simulink model "V2"  (R2024b)
settings: Solver=ode4  StartTime=0.0  StopTime=EXP.stop_time  FixedStep=EXP.physics_step  RelTol=1e-3
PostLoadFcn:
  | addpath(fullfile(fileparts(get_param(bdroot,'FileName')),'simulink_config')); v2_initialize_model(bdroot);
InitFcn:
  | addpath(fullfile(fileparts(get_param(bdroot,'FileName')),'simulink_config')); v2_initialize_model(bdroot);
model workspace (MAT data in the model file):
  CTRL.sample_time = 0.0025
  CTRL.position.Kp = [2.5 2.5 3.4]
  CTRL.position.Ki = [0 0 0]
  CTRL.position.Kd = [0 0 0]
  CTRL.position.integral_limit = [0.3 0.3 0.3]
  CTRL.position.output_limit = [10 10 100]
  CTRL.position.derivative_cutoff_hz = 10
  CTRL.position.velocity_ff.enable = 0
  CTRL.position.velocity_ff.cutoff_hz = 10
  CTRL.velocity.Kp = [3.5 3.5 8]
  CTRL.velocity.Ki = [0.12 0.12 2.5]
  CTRL.velocity.Kd = [0.08 0.08 0.07]
  CTRL.velocity.integral_limit = [10 10 10]
  CTRL.velocity.output_limit = [1000 1000 1000]
  CTRL.velocity.derivative_cutoff_hz = 10
  CTRL.velocity.gravity_comp.enable = 1
  CTRL.attitude.Kp = [10 10 4.5]
  CTRL.attitude.Ki = [0 0 0]
  CTRL.attitude.Kd = [0.05 0.05 0.01]
  CTRL.attitude.integral_limit = [0.2 0.2 0.2]
  CTRL.attitude.output_limit = [3.84 3.84 3.49]
  CTRL.attitude.derivative_cutoff_hz = 15
  CTRL.rate.Kp = [2.2 2.2 1.6]
  CTRL.rate.Ki = [0 0 0]
  CTRL.rate.Kd = [0.04 0.04 0.02]
  CTRL.rate.integral_limit = [0.4 0.4 0.4]
  CTRL.rate.output_limit = [4 4 3]
  CTRL.rate.derivative_cutoff_hz = 20
  CTRL.rate.gyroscopic_ff.enable = 1
  CTRL.force_limit = [30 30 100]
  CTRL.torque_limit = [5 5 4]
  CTRL.nominal.mass = 6
  CTRL.nominal.gravity = 9.80665
  CTRL.nominal.inertia = [0.2  0  0; 0  0.2  0; 0  0  0.2]
  CTRL.nominal.geometry.arm_length = 0.4
  CTRL.nominal.geometry.rotor_z = -0.015
  CTRL.nominal.geometry.radial_xy = [0.707106781187  -0.707106781187  -0.707106781187  0.707106781187; 0.707106781187  0.707106781187  -0.707106781187  -0.707106781187]
  CTRL.nominal.geometry.tangent = [0.707106781187  0.707106781187  -0.707106781187  -0.707106781187; -0.707106781187  0.707106781187  0.707106781187  -0.707106781187; 0  0  0  0]
  CTRL.nominal.geometry.spin = [-1 1 -1 1]
  CTRL.nominal.propeller.b_over_k = 0.01
  CTRL.nominal.propeller.reaction_torque_ratio = 0.01
  CTRL.nominal.propeller.max_thrust = 200
  CTRL.nominal.servo_limit = 1
  CTRL.allocator.yaw_split_cutoff_hz = 0.5
  CTRL.allocator.yaw_reaction_limit = 0.6
  CTRL.allocator.regularization = 1e-08
  CTRL.dob.enable = 1
  CTRL.dob.cutoff_rad_s = 2
  CTRL.dob.estimate_limit = [3 3 3]
  CTRL.moce.enable = 0
  CTRL.moce.gamma = [7e-06 7e-06 0.00015]
  CTRL.moce.initial_com = [0 0 0]
  CTRL.moce.offset_limit = [0.15 0.15 0.15]
  CTRL.moce.rate_limit = [0.02 0.02 0.02]
  CTRL.moce.min_force = 5
  CTRL.moce.estimate_z = 0
  CTRL.moce.min_horizontal_force = 0.1
  CTRL.moce.force_cutoff_rad_s = 2
  CTRL.moce.output_tau_s = 0.15
  EXP.command.position = [0 0 1]
  EXP.command.position_mode = 0
  EXP.command.position_sine_amplitude = [0 -10 0]
  EXP.command.position_sine_rad_s = [0 0.5 0]
  EXP.command.position_sine_phase = [0 0 0]
  EXP.command.position_start_s = 10
  EXP.command.attitude = [0 0 0]
  EXP.command.attitude_sine_enable = [0 0 0]
  EXP.command.attitude_sine_amplitude = [0.2 -0.2 -1]
  EXP.command.attitude_sine_rad_s = [0.4 0.4 0.2]
  EXP.command.attitude_sine_phase = [0 0 0]
  EXP.payload.mass = 0
  EXP.payload.position = [0 0 0]
  EXP.initial.position = [0 0 0]
  EXP.initial.velocity = [0 0 0]
  EXP.initial.attitude = [0 0 0]
  EXP.initial.body_rate = [0 0 0]
  EXP.seed = 1
  EXP.stop_time = 10
  EXP.physics_step = 0.00125
  PLANT.vehicle.mass = 6
  PLANT.vehicle.com = [0.01 0.005 0.001]
  PLANT.vehicle.inertia = [0.3  0  0; 0  0.3  0; 0  0  0.4]
  PLANT.gravity = 9.80665
  PLANT.geometry.arm_length = 0.4
  PLANT.geometry.rotor_z = -0.015
  PLANT.geometry.radial_xy = [0.707106781187  -0.707106781187  -0.707106781187  0.707106781187; 0.707106781187  0.707106781187  -0.707106781187  -0.707106781187]
  PLANT.geometry.tangent = [0.707106781187  0.707106781187  -0.707106781187  -0.707106781187; -0.707106781187  0.707106781187  0.707106781187  -0.707106781187; 0  0  0  0]
  PLANT.geometry.spin = [-1 1 -1 1]
  PLANT.propeller.b_over_k = 0.01
  PLANT.propeller.reaction_torque_ratio = 0.01
  PLANT.propeller.time_constant_s = 0.01
  PLANT.propeller.delay_s = 0
  PLANT.propeller.effectiveness = [0.8; 0.8; 0.8; 0.8]
  PLANT.propeller.max_thrust = 200
  PLANT.propeller.initial_thrust = [0; 0; 0; 0]
  PLANT.servo.time_constant_s = 0.0333333333333
  PLANT.servo.delay_s = 0
  PLANT.servo.dc_gain = 1
  PLANT.servo.limit_rad = 1
  PLANT.servo.initial_angle = [0; 0; 0; 0]
  PLANT.derived.mass = 6
  PLANT.derived.com = [0.01; 0.005; 0.001]
  PLANT.derived.inertia = [0.3  0  0; 0  0.3  0; 0  0  0.4]
  SENSOR.position.enable = 0
  SENSOR.position.noise_std = [0.00019 0.00022 0.00017]
  SENSOR.position.bias = [0 0 0]
  SENSOR.velocity.enable = 0
  SENSOR.velocity.noise_std = [0.00473 0.005 0.00368]
  SENSOR.velocity.bias = [0 0 0]
  SENSOR.attitude.enable = 0
  SENSOR.attitude.noise_std = [0.00071 0.00067 0.00044]
  SENSOR.attitude.bias = [0 0 0]
  SENSOR.gyro.enable = 0
  SENSOR.gyro.noise_std = [0.0236 0.0215 0.0174]
  SENSOR.gyro.bias = [0 0 0]
  SENSOR.delay_s = 0
settings Model: Creator=seosuk  LastModifiedBy=seosuk
settings DataIOCC: SaveOutput=off
settings DebuggingCC: AlgebraicLoopMsg=error

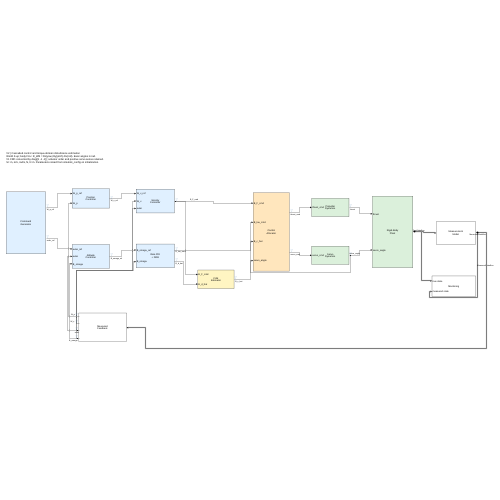
[thumbnail: Simulink's stored preview of the top-level diagram]
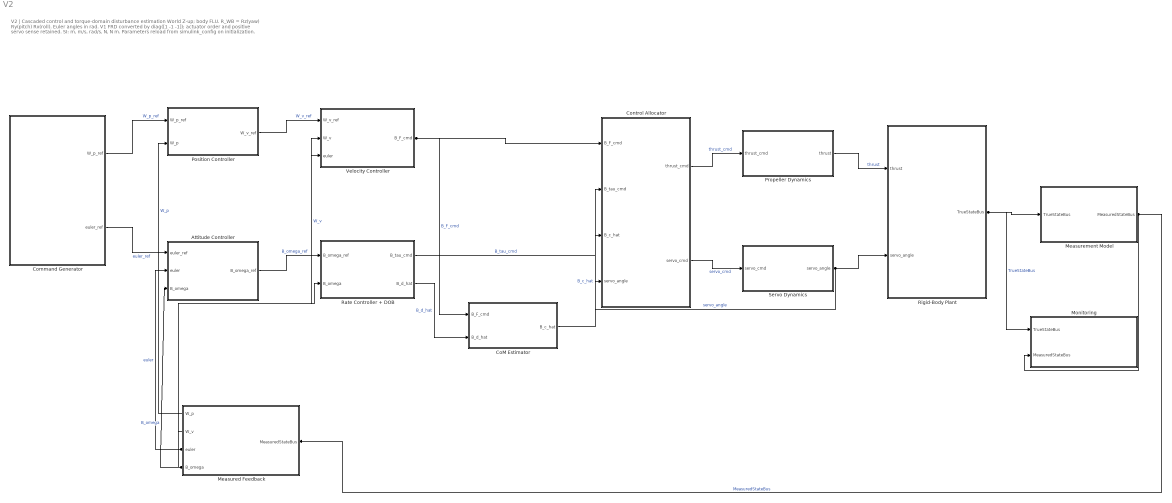
== system V2 ==
  note: V2 | Cascaded control and torque-domain disturbance estimation
      | World Z-up; body FLU. R_WB = Rz(yaw) Ry(pitch) Rx(roll). Euler angles in rad.
      | V1 FRD converted by diag([1 -1 -1]); actuator order and positive servo sense retained.
      | SI: m, m/s, rad/s, N, N m. Parameters reload from simulink_config on initialization.
  Attitude Controller : Subsystem
      mask Display:
      | disp(sprintf('Attitude\nController'));
      | port_label('input',1,'euler_ref');
      | port_label('input',2,'euler');
      | port_label('input',3,'B_omega');
  CoM Estimator : Subsystem
      mask Display:
      | disp(sprintf('CoM\nEstimator'));
      | port_label('input',1,'B_F_cmd');
      | port_label('input',2,'B_d_hat');
  Command Generator : Subsystem
      mask Display: disp(sprintf('Command\nGenerator'));
  Control Allocator : Subsystem
      mask Display:
      | disp(sprintf('Control\nAllocator'));
      | port_label('input',1,'B_F_cmd');
      | port_label('input',2,'B_tau_cmd');
      | port_label('input',3,'B_c_hat');
      | port_label('input',4,'servo_angle');
  Measured Feedback : Subsystem
      mask Display: disp(sprintf('Measured\nFeedback'));
  Measurement Model : Subsystem
      mask Display: disp(sprintf('Measurement\nModel'));
  Monitoring : Subsystem
      mask Display:
      | disp(sprintf('Monitoring'));
      | port_label('input',1,'true state');
      | port_label('input',2,'measured state');
  Position Controller : Subsystem
      mask Display:
      | disp(sprintf('Position\nController'));
      | port_label('input',1,'W_p_ref');
      | port_label('input',2,'W_p');
  Propeller Dynamics : Subsystem
      mask Display:
      | disp(sprintf('Propeller\nDynamics'));
      | port_label('input',1,'thrust_cmd');
  Rate Controller + DOB : Subsystem
      mask Display:
      | disp(sprintf('Rate PID\n+ DOB'));
      | port_label('input',1,'B_omega_ref');
      | port_label('input',2,'B_omega');
  Rigid-Body Plant : Subsystem
      mask Display:
      | disp(sprintf('Rigid-Body\nPlant'));
      | port_label('input',1,'thrust');
      | port_label('input',2,'servo_angle');
  Servo Dynamics : Subsystem
      mask Display:
      | disp(sprintf('Servo\nDynamics'));
      | port_label('input',1,'servo_cmd');
  Velocity Controller : Subsystem
      mask Display:
      | disp(sprintf('Velocity\nController'));
      | port_label('input',1,'W_v_ref');
      | port_label('input',2,'W_v');
      | port_label('input',3,'euler');
  wires:
  Command Generator/1(W_p_ref) -> Position Controller/1(W_p_ref)  "W_p_ref"
  Command Generator/2(euler_ref) -> Attitude Controller/1(euler_ref)  "euler_ref"
  Position Controller/1(W_v_ref) -> Velocity Controller/1(W_v_ref)  "W_v_ref"
  Velocity Controller/1(B_F_cmd) -> Control Allocator/1(B_F_cmd), CoM Estimator/1(B_F_cmd)  "B_F_cmd"
  Attitude Controller/1(B_omega_ref) -> Rate Controller + DOB/1(B_omega_ref)  "B_omega_ref"
  Rate Controller + DOB/1(B_tau_cmd) -> Control Allocator/2(B_tau_cmd)  "B_tau_cmd"
  Rate Controller + DOB/2(B_d_hat) -> CoM Estimator/2(B_d_hat)  "B_d_hat"
  CoM Estimator/1(B_c_hat) -> Control Allocator/3(B_c_hat)  "B_c_hat"
  Control Allocator/1(thrust_cmd) -> Propeller Dynamics/1(thrust_cmd)  "thrust_cmd"
  Control Allocator/2(servo_cmd) -> Servo Dynamics/1(servo_cmd)  "servo_cmd"
  Propeller Dynamics/1(thrust) -> Rigid-Body Plant/1(thrust)  "thrust"
  Servo Dynamics/1(servo_angle) -> Rigid-Body Plant/2(servo_angle), Control Allocator/4(servo_angle)  "servo_angle"
  Rigid-Body Plant/1(TrueStateBus) -> Measurement Model/1(TrueStateBus), Monitoring/1(TrueStateBus)  "TrueStateBus"
  Measurement Model/1(MeasuredStateBus) -> Monitoring/2(MeasuredStateBus), Measured Feedback/1(MeasuredStateBus)  "MeasuredStateBus"
  Measured Feedback/1(W_p) -> Position Controller/2(W_p)  "W_p"
  Measured Feedback/2(W_v) -> Velocity Controller/2(W_v)  "W_v"
  Measured Feedback/3(euler) -> Velocity Controller/3(euler), Attitude Controller/2(euler)  "euler"
  Measured Feedback/4(B_omega) -> Attitude Controller/3(B_omega), Rate Controller + DOB/2(B_omega)  "B_omega"

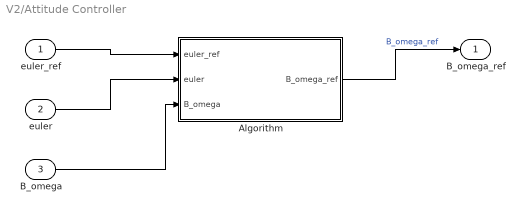
== system V2/Attitude Controller ==
  euler_ref : Inport  PortDimensions=[3 1]
  euler : Inport  Port=2  PortDimensions=[3 1]
  B_omega : Inport  Port=3  PortDimensions=[3 1]
  Algorithm : MATLAB Function  TreatAsAtomicUnit=on
  B_omega_ref : Outport
  wires:
  euler_ref/1 -> Algorithm/1(euler_ref)
  euler/1 -> Algorithm/2(euler)
  B_omega/1 -> Algorithm/3(B_omega)
  Algorithm/1(B_omega_ref) -> B_omega_ref/1  "B_omega_ref"

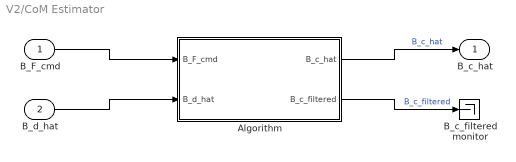
== system V2/CoM Estimator ==
  B_F_cmd : Inport  PortDimensions=[3 1]
  B_d_hat : Inport  Port=2  PortDimensions=[3 1]
  Algorithm : MATLAB Function  TreatAsAtomicUnit=on
  B_c_filtered monitor : Terminator
  B_c_hat : Outport
  wires:
  B_F_cmd/1 -> Algorithm/1(B_F_cmd)
  B_d_hat/1 -> Algorithm/2(B_d_hat)
  Algorithm/1(B_c_hat) -> B_c_hat/1  "B_c_hat"
  Algorithm/2(B_c_filtered) -> B_c_filtered monitor/1  "B_c_filtered"

== system V2/Command Generator ==
  Algorithm : MATLAB Function  TreatAsAtomicUnit=on
  Experiment time : Clock
  W_p_ref : Outport
  euler_ref : Outport  Port=2
  wires:
  Algorithm/1(W_p_ref) -> W_p_ref/1  "W_p_ref"
  Algorithm/2(euler_ref) -> euler_ref/1  "euler_ref"
  Experiment time/1 -> Algorithm/1(t)

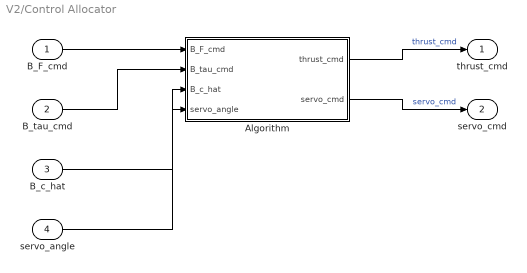
== system V2/Control Allocator ==
  B_F_cmd : Inport  PortDimensions=[3 1]
  B_tau_cmd : Inport  Port=2  PortDimensions=[3 1]
  B_c_hat : Inport  Port=3  PortDimensions=[3 1]
  servo_angle : Inport  Port=4  PortDimensions=[4 1]
  Algorithm : MATLAB Function  TreatAsAtomicUnit=on
  thrust_cmd : Outport
  servo_cmd : Outport  Port=2
  wires:
  B_F_cmd/1 -> Algorithm/1(B_F_cmd)
  B_tau_cmd/1 -> Algorithm/2(B_tau_cmd)
  B_c_hat/1 -> Algorithm/3(B_c_hat)
  servo_angle/1 -> Algorithm/4(servo_angle)
  Algorithm/1(thrust_cmd) -> thrust_cmd/1  "thrust_cmd"
  Algorithm/2(servo_cmd) -> servo_cmd/1  "servo_cmd"

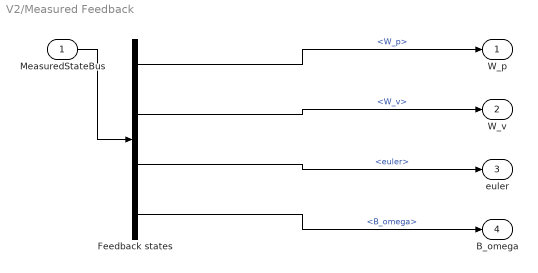
== system V2/Measured Feedback ==
  MeasuredStateBus : Inport
  Feedback states : BusSelector  OutputSignals=W_p,W_v,euler,B_omega
  W_p : Outport
  W_v : Outport  Port=2
  euler : Outport  Port=3
  B_omega : Outport  Port=4
  wires:
  MeasuredStateBus/1 -> Feedback states/1
  Feedback states/1 -> W_p/1  "<W_p>"
  Feedback states/2 -> W_v/1  "<W_v>"
  Feedback states/3 -> euler/1  "<euler>"
  Feedback states/4 -> B_omega/1  "<B_omega>"

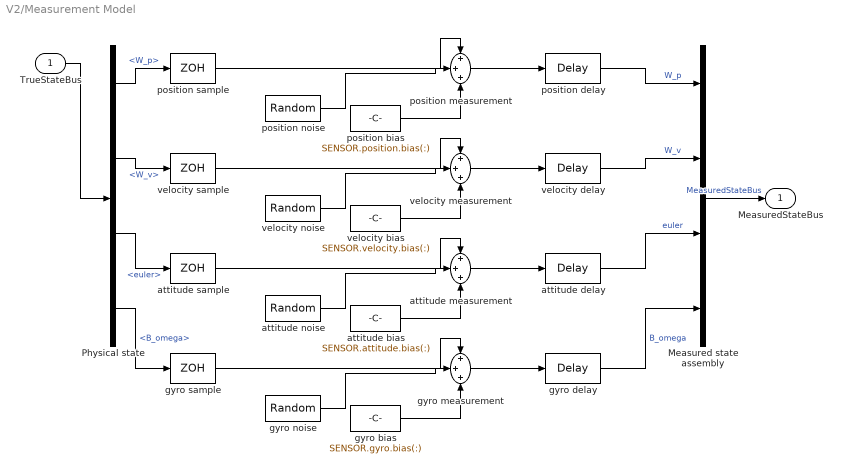
== system V2/Measurement Model ==
  TrueStateBus : Inport
  Measured state assembly : BusCreator  Inputs=4
  Physical state : BusSelector  OutputSignals=W_p,W_v,euler,B_omega
  attitude bias : Constant  Value=SENSOR.attitude.bias(:)
  attitude delay : TransportDelay  DelayTime=SENSOR.delay_s  TransDelayFeedthrough=on
  attitude measurement : Sum  Inputs=+++
  attitude noise : RandomNumber  Mean=[0;0;0]  Variance=double(SENSOR.attitude.enable)*SENSOR.attitude.noise_std(:).^2  Seed=EXP.seed+303  SampleTime=CTRL.sample_time
  attitude sample : ZeroOrderHold  SampleTime=CTRL.sample_time
  gyro bias : Constant  Value=SENSOR.gyro.bias(:)
  gyro delay : TransportDelay  DelayTime=SENSOR.delay_s  TransDelayFeedthrough=on
  gyro measurement : Sum  Inputs=+++
  gyro noise : RandomNumber  Mean=[0;0;0]  Variance=double(SENSOR.gyro.enable)*SENSOR.gyro.noise_std(:).^2  Seed=EXP.seed+404  SampleTime=CTRL.sample_time
  gyro sample : ZeroOrderHold  SampleTime=CTRL.sample_time
  position bias : Constant  Value=SENSOR.position.bias(:)
  position delay : TransportDelay  DelayTime=SENSOR.delay_s  TransDelayFeedthrough=on
  position measurement : Sum  Inputs=+++
  position noise : RandomNumber  Mean=[0;0;0]  Variance=double(SENSOR.position.enable)*SENSOR.position.noise_std(:).^2  Seed=EXP.seed+101  SampleTime=CTRL.sample_time
  position sample : ZeroOrderHold  SampleTime=CTRL.sample_time
  velocity bias : Constant  Value=SENSOR.velocity.bias(:)
  velocity delay : TransportDelay  DelayTime=SENSOR.delay_s  TransDelayFeedthrough=on
  velocity measurement : Sum  Inputs=+++
  velocity noise : RandomNumber  Mean=[0;0;0]  Variance=double(SENSOR.velocity.enable)*SENSOR.velocity.noise_std(:).^2  Seed=EXP.seed+202  SampleTime=CTRL.sample_time
  velocity sample : ZeroOrderHold  SampleTime=CTRL.sample_time
  MeasuredStateBus : Outport
  wires:
  TrueStateBus/1 -> Physical state/1
  Physical state/1 -> position sample/1  "<W_p>"
  position sample/1 -> position measurement/1
  position noise/1 -> position measurement/2
  position bias/1 -> position measurement/3
  position measurement/1 -> position delay/1
  position delay/1 -> Measured state assembly/1  "W_p"
  Physical state/2 -> velocity sample/1  "<W_v>"
  velocity sample/1 -> velocity measurement/1
  velocity noise/1 -> velocity measurement/2
  velocity bias/1 -> velocity measurement/3
  velocity measurement/1 -> velocity delay/1
  velocity delay/1 -> Measured state assembly/2  "W_v"
  Physical state/3 -> attitude sample/1  "<euler>"
  attitude sample/1 -> attitude measurement/1
  attitude noise/1 -> attitude measurement/2
  attitude bias/1 -> attitude measurement/3
  attitude measurement/1 -> attitude delay/1
  attitude delay/1 -> Measured state assembly/3  "euler"
  Physical state/4 -> gyro sample/1  "<B_omega>"
  gyro sample/1 -> gyro measurement/1
  gyro noise/1 -> gyro measurement/2
  gyro bias/1 -> gyro measurement/3
  gyro measurement/1 -> gyro delay/1
  gyro delay/1 -> Measured state assembly/4  "B_omega"
  Measured state assembly/1 -> MeasuredStateBus/1  "MeasuredStateBus"

== system V2/Monitoring ==
  note: Read-only diagnostics. All named control/actuator signals are logged to logsout.
      | Use Simulation Data Inspector or out.logsout. PID/nominal torque and filtered CoM
      | are logged inside their producing subsystems, with no diagnostic feedback.
  TrueStateBus : Inport
  MeasuredStateBus : Inport  Port=2
  Measured state : Scope
  True state : Scope
  wires:
  TrueStateBus/1 -> True state/1
  MeasuredStateBus/1 -> Measured state/1

== system V2/Position Controller ==
  W_p_ref : Inport  PortDimensions=[3 1]
  W_p : Inport  Port=2  PortDimensions=[3 1]
  Algorithm : MATLAB Function  TreatAsAtomicUnit=on
  W_v_ref : Outport
  wires:
  W_p_ref/1 -> Algorithm/1(W_p_ref)
  W_p/1 -> Algorithm/2(W_p)
  Algorithm/1(W_v_ref) -> W_v_ref/1  "W_v_ref"

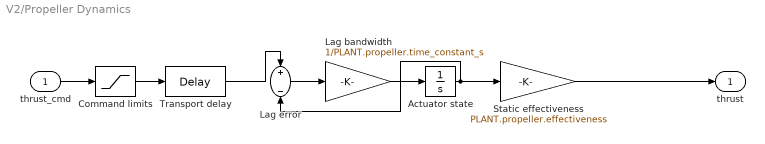
== system V2/Propeller Dynamics ==
  thrust_cmd : Inport  PortDimensions=[4 1]
  Actuator state : Integrator  InitialCondition=PLANT.propeller.initial_thrust
  Command limits : Saturate  UpperLimit=PLANT.propeller.max_thrust  LowerLimit=0
  Lag bandwidth : Gain  Gain=1/PLANT.propeller.time_constant_s
  Lag error : Sum  Inputs=+-
  Static effectiveness : Gain  Gain=PLANT.propeller.effectiveness
  Transport delay : TransportDelay  DelayTime=PLANT.propeller.delay_s  TransDelayFeedthrough=on
  thrust : Outport
  wires:
  thrust_cmd/1 -> Command limits/1
  Command limits/1 -> Transport delay/1
  Transport delay/1 -> Lag error/1
  Actuator state/1 -> Lag error/2, Static effectiveness/1
  Lag error/1 -> Lag bandwidth/1
  Lag bandwidth/1 -> Actuator state/1
  Static effectiveness/1 -> thrust/1

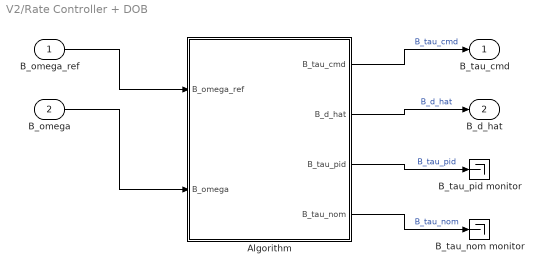
== system V2/Rate Controller + DOB ==
  B_omega_ref : Inport  PortDimensions=[3 1]
  B_omega : Inport  Port=2  PortDimensions=[3 1]
  Algorithm : MATLAB Function  TreatAsAtomicUnit=on
  B_tau_nom monitor : Terminator
  B_tau_pid monitor : Terminator
  B_tau_cmd : Outport
  B_d_hat : Outport  Port=2
  wires:
  B_omega_ref/1 -> Algorithm/1(B_omega_ref)
  B_omega/1 -> Algorithm/2(B_omega)
  Algorithm/1(B_tau_cmd) -> B_tau_cmd/1  "B_tau_cmd"
  Algorithm/2(B_d_hat) -> B_d_hat/1  "B_d_hat"
  Algorithm/3(B_tau_pid) -> B_tau_pid monitor/1  "B_tau_pid"
  Algorithm/4(B_tau_nom) -> B_tau_nom monitor/1  "B_tau_nom"

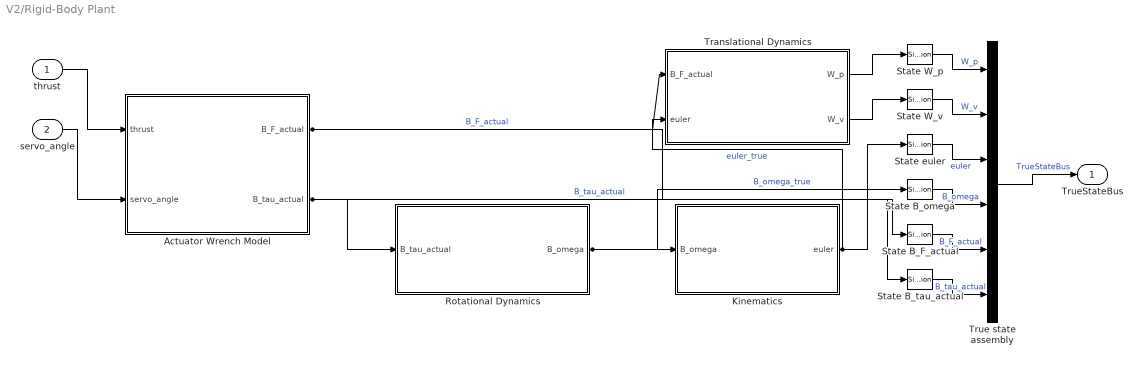
== system V2/Rigid-Body Plant ==
  thrust : Inport
  servo_angle : Inport  Port=2
  Actuator Wrench Model : Subsystem
  Kinematics : Subsystem
  Rotational Dynamics : Subsystem
  State B_F_actual : SignalConversion  OverrideOpt=off
  State B_omega : SignalConversion  OverrideOpt=off
  State B_tau_actual : SignalConversion  OverrideOpt=off
  State W_p : SignalConversion  OverrideOpt=off
  State W_v : SignalConversion  OverrideOpt=off
  State euler : SignalConversion  OverrideOpt=off
  Translational Dynamics : Subsystem
  True state assembly : BusCreator  Inputs=6
  TrueStateBus : Outport
  wires:
  thrust/1 -> Actuator Wrench Model/1(thrust)
  servo_angle/1 -> Actuator Wrench Model/2(servo_angle)
  Actuator Wrench Model/1(B_F_actual) -> Translational Dynamics/1(B_F_actual), State B_F_actual/1  "B_F_actual"
  Actuator Wrench Model/2(B_tau_actual) -> Rotational Dynamics/1(B_tau_actual), State B_tau_actual/1  "B_tau_actual"
  Rotational Dynamics/1(B_omega) -> Kinematics/1(B_omega), State B_omega/1  "B_omega_true"
  Kinematics/1(euler) -> Translational Dynamics/2(euler), State euler/1  "euler_true"
  Translational Dynamics/1(W_p) -> State W_p/1
  State W_p/1 -> True state assembly/1  "W_p"
  Translational Dynamics/2(W_v) -> State W_v/1
  State W_v/1 -> True state assembly/2  "W_v"
  State euler/1 -> True state assembly/3  "euler"
  State B_omega/1 -> True state assembly/4  "B_omega"
  State B_F_actual/1 -> True state assembly/5  "B_F_actual"
  State B_tau_actual/1 -> True state assembly/6  "B_tau_actual"
  True state assembly/1 -> TrueStateBus/1  "TrueStateBus"

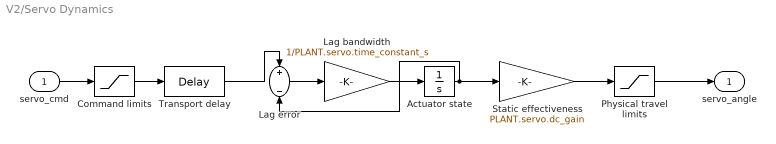
== system V2/Servo Dynamics ==
  servo_cmd : Inport  PortDimensions=[4 1]
  Actuator state : Integrator  InitialCondition=PLANT.servo.initial_angle
  Command limits : Saturate  UpperLimit=PLANT.servo.limit_rad  LowerLimit=-PLANT.servo.limit_rad
  Lag bandwidth : Gain  Gain=1/PLANT.servo.time_constant_s
  Lag error : Sum  Inputs=+-
  Physical travel limits : Saturate  UpperLimit=PLANT.servo.limit_rad  LowerLimit=-PLANT.servo.limit_rad
  Static effectiveness : Gain  Gain=PLANT.servo.dc_gain
  Transport delay : TransportDelay  DelayTime=PLANT.servo.delay_s  TransDelayFeedthrough=on
  servo_angle : Outport
  wires:
  servo_cmd/1 -> Command limits/1
  Command limits/1 -> Transport delay/1
  Transport delay/1 -> Lag error/1
  Actuator state/1 -> Lag error/2, Static effectiveness/1
  Lag error/1 -> Lag bandwidth/1
  Lag bandwidth/1 -> Actuator state/1
  Static effectiveness/1 -> Physical travel limits/1
  Physical travel limits/1 -> servo_angle/1

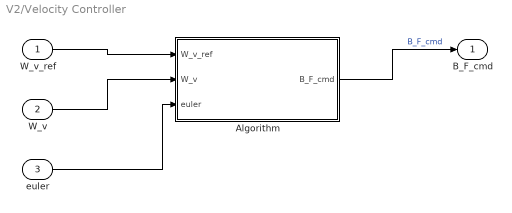
== system V2/Velocity Controller ==
  W_v_ref : Inport  PortDimensions=[3 1]
  W_v : Inport  Port=2  PortDimensions=[3 1]
  euler : Inport  Port=3  PortDimensions=[3 1]
  Algorithm : MATLAB Function  TreatAsAtomicUnit=on
  B_F_cmd : Outport
  wires:
  W_v_ref/1 -> Algorithm/1(W_v_ref)
  W_v/1 -> Algorithm/2(W_v)
  euler/1 -> Algorithm/3(euler)
  Algorithm/1(B_F_cmd) -> B_F_cmd/1  "B_F_cmd"

== system V2/Rigid-Body Plant/Actuator Wrench Model ==
  thrust : Inport  PortDimensions=[4 1]
  servo_angle : Inport  Port=2  PortDimensions=[4 1]
  Algorithm : MATLAB Function  TreatAsAtomicUnit=on
  B_F_actual : Outport
  B_tau_actual : Outport  Port=2
  wires:
  thrust/1 -> Algorithm/1(thrust)
  servo_angle/1 -> Algorithm/2(servo_angle)
  Algorithm/1(B_F_actual) -> B_F_actual/1  "B_F_actual"
  Algorithm/2(B_tau_actual) -> B_tau_actual/1  "B_tau_actual"

== system V2/Rigid-Body Plant/Kinematics ==
  B_omega : Inport
  Euler angle rates : Subsystem
  Euler attitude : Integrator  InitialCondition=EXP.initial.attitude(:)
  euler : Outport
  wires:
  B_omega/1 -> Euler angle rates/2(B_omega)
  Euler angle rates/1(euler_dot) -> Euler attitude/1
  Euler attitude/1 -> Euler angle rates/1(euler), euler/1

== system V2/Rigid-Body Plant/Rotational Dynamics ==
  B_tau_actual : Inport
  Body rate : Integrator  InitialCondition=EXP.initial.body_rate(:)
  Euler rigid body equation : Subsystem
  B_omega : Outport
  wires:
  B_tau_actual/1 -> Euler rigid body equation/1(B_tau_actual)
  Euler rigid body equation/1(B_omega_dot) -> Body rate/1
  Body rate/1 -> Euler rigid body equation/2(B_omega), B_omega/1

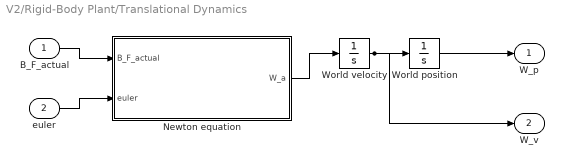
== system V2/Rigid-Body Plant/Translational Dynamics ==
  B_F_actual : Inport
  euler : Inport  Port=2
  Newton equation : Subsystem
  World position : Integrator  InitialCondition=EXP.initial.position(:)
  World velocity : Integrator  InitialCondition=EXP.initial.velocity(:)
  W_p : Outport
  W_v : Outport  Port=2
  wires:
  B_F_actual/1 -> Newton equation/1(B_F_actual)
  euler/1 -> Newton equation/2(euler)
  Newton equation/1(W_a) -> World velocity/1
  World velocity/1 -> World position/1, W_v/1
  World position/1 -> W_p/1

== system V2/Rigid-Body Plant/Kinematics/Euler angle rates ==
  euler : Inport  PortDimensions=[3 1]
  B_omega : Inport  Port=2  PortDimensions=[3 1]
  Algorithm : MATLAB Function  TreatAsAtomicUnit=on
  euler_dot : Outport
  wires:
  euler/1 -> Algorithm/1(euler)
  B_omega/1 -> Algorithm/2(B_omega)
  Algorithm/1(euler_dot) -> euler_dot/1  "euler_dot"

== system V2/Rigid-Body Plant/Rotational Dynamics/Euler rigid body equation ==
  B_tau_actual : Inport  PortDimensions=[3 1]
  B_omega : Inport  Port=2  PortDimensions=[3 1]
  Algorithm : MATLAB Function  TreatAsAtomicUnit=on
  B_omega_dot : Outport
  wires:
  B_tau_actual/1 -> Algorithm/1(B_tau_actual)
  B_omega/1 -> Algorithm/2(B_omega)
  Algorithm/1(B_omega_dot) -> B_omega_dot/1  "B_omega_dot"

== system V2/Rigid-Body Plant/Translational Dynamics/Newton equation ==
  B_F_actual : Inport  PortDimensions=[3 1]
  euler : Inport  Port=2  PortDimensions=[3 1]
  Algorithm : MATLAB Function  TreatAsAtomicUnit=on
  W_a : Outport
  wires:
  B_F_actual/1 -> Algorithm/1(B_F_actual)
  euler/1 -> Algorithm/2(euler)
  Algorithm/1(W_a) -> W_a/1  "W_a"

== matlab function V2/Rigid-Body Plant/Kinematics/Euler angle rates/Algorithm ==
  data: euler input; euler_dot output; B_omega input
function euler_dot = v2_kinematics(euler,B_omega)
%#codegen
% V1 Euler kinematics; Euler representation is singular at pitch +/-pi/2.
s=sin(euler(1)); c=cos(euler(1)); ct=cos(euler(2));
assert(abs(ct)>1e-6,'Euler pitch singularity');
euler_dot=[1 s*tan(euler(2)) c*tan(euler(2));0 c -s;0 s/ct c/ct]*B_omega;
end

== matlab function V2/Rigid-Body Plant/Translational Dynamics/Newton equation/Algorithm ==
  data: B_F_actual input; W_a output; euler input; PLANT parameter
function W_a = v2_translation_dynamics(B_F_actual,euler,PLANT)
%#codegen
W_a=v2_rotation(euler)*B_F_actual/PLANT.derived.mass-[0;0;PLANT.gravity];
end

== matlab function V2/Position Controller/Algorithm ==
  settings: updateMethod=DISCRETE  sampleTime=CTRL.sample_time
  data: W_p_ref input; W_v_ref output; W_p input; CTRL parameter
function W_v_ref = v2_position(W_p_ref,W_p,CTRL)
%#codegen
persistent integral derivative previous previous_ref ff
if isempty(integral)
    integral=zeros(3,1); derivative=zeros(3,1); previous=W_p;
    previous_ref=W_p_ref; ff=zeros(3,1);
end
dt=CTRL.sample_time;
ff=ff+(1-exp(-2*pi*CTRL.position.velocity_ff.cutoff_hz*dt))*((W_p_ref-previous_ref)/dt-ff);
feedforward=zeros(3,1);
if CTRL.position.velocity_ff.enable, feedforward=ff; end
[W_v_ref,integral,derivative]=v2_pid(W_p_ref-W_p,(W_p-previous)/dt, ...
    integral,derivative,CTRL.position,dt,feedforward);
previous=W_p; previous_ref=W_p_ref;
end

== matlab function V2/Command Generator/Algorithm ==
  data: t input; W_p_ref output; euler_ref output; EXP parameter
function [W_p_ref,euler_ref] = v2_command(t,EXP)
%#codegen
W_p_ref=EXP.command.position(:);
if EXP.command.position_mode==1 && t>EXP.command.position_start_s
    W_p_ref=W_p_ref+EXP.command.position_sine_amplitude(:).* ...
        sin(EXP.command.position_sine_rad_s(:)*t+EXP.command.position_sine_phase(:));
end
euler_ref=EXP.command.attitude(:)+double(EXP.command.attitude_sine_enable(:)).* ...
    EXP.command.attitude_sine_amplitude(:).*sin(EXP.command.attitude_sine_rad_s(:)*t+EXP.command.attitude_sine_phase(:));
end

== matlab function V2/Velocity Controller/Algorithm ==
  settings: updateMethod=DISCRETE  sampleTime=CTRL.sample_time
  data: W_v_ref input; B_F_cmd output; W_v input; euler input; CTRL parameter
function B_F_cmd = v2_velocity(W_v_ref,W_v,euler,CTRL)
%#codegen
persistent integral derivative previous
if isempty(integral), integral=zeros(3,1); derivative=zeros(3,1); previous=W_v; end
dt=CTRL.sample_time;
[a,integral,derivative]=v2_pid(W_v_ref-W_v,(W_v-previous)/dt,integral,derivative,CTRL.velocity,dt,zeros(3,1));
if CTRL.velocity.gravity_comp.enable, a(3)=a(3)+CTRL.nominal.gravity; end
W_F_cmd=CTRL.nominal.mass*a;
W_F_cmd(3)=max(0,W_F_cmd(3)); % C++ nonnegative vertical thrust demand
B_F_cmd=v2_bound(v2_rotation(euler)'*W_F_cmd,CTRL.force_limit);
previous=W_v;
end

== matlab function V2/Attitude Controller/Algorithm ==
  settings: updateMethod=DISCRETE  sampleTime=CTRL.sample_time
  data: euler_ref input; B_omega_ref output; euler input; B_omega input; CTRL parameter
function B_omega_ref = v2_attitude(euler_ref,euler,B_omega,CTRL)
%#codegen
persistent integral derivative
if isempty(integral), integral=zeros(3,1); derivative=zeros(3,1); end
error=v2_rotvec(v2_rotation(euler)'*v2_rotation(euler_ref));
[B_omega_ref,integral,derivative]=v2_pid(error,B_omega,integral,derivative,CTRL.attitude,CTRL.sample_time,zeros(3,1));
end

== matlab function V2/Rate Controller + DOB/Algorithm ==
  settings: updateMethod=DISCRETE  sampleTime=CTRL.sample_time
  data: B_omega_ref input; B_tau_cmd output; B_omega input; B_d_hat output; B_tau_pid output; B_tau_nom output; CTRL parameter
function [B_tau_cmd,B_d_hat,B_tau_pid,B_tau_nom] = v2_rate_dob(B_omega_ref,B_omega,CTRL)
%#codegen
persistent integral derivative previous rate_state torque_state estimate
if isempty(integral)
    integral=zeros(3,1); derivative=zeros(3,1); previous=B_omega;
    rate_state=[zeros(1,3);B_omega(:)'/CTRL.dob.cutoff_rad_s^2];
    torque_state=zeros(2,3); estimate=zeros(3,1);
end
dt=CTRL.sample_time; J=CTRL.nominal.inertia;
[B_tau_pid,integral,derivative]=v2_pid(B_omega_ref-B_omega,(B_omega-previous)/dt, ...
    integral,derivative,CTRL.rate,dt,zeros(3,1));
gyro=cross(B_omega,J*B_omega);
B_tau_nom=B_tau_pid;
if CTRL.rate.gyroscopic_ff.enable, B_tau_nom=B_tau_nom+gyro; end
B_d_hat=zeros(3,1);
if CTRL.dob.enable
    % C++ predictor uses previous estimate, bounds torque, then removes actual
    % nominal gyroscopic torque irrespective of feed-forward switch.
    effective=v2_bound(B_tau_nom-estimate,CTRL.torque_limit)-gyro;
    [rate_state,~,dq]=v2_q(rate_state,B_omega,CTRL.dob.cutoff_rad_s,dt);
    [torque_state,qt,~]=v2_q(torque_state,effective,CTRL.dob.cutoff_rad_s,dt);
    B_d_hat=v2_bound(J*dq-qt,CTRL.dob.estimate_limit);
end
estimate=B_d_hat;
B_tau_cmd=v2_bound(B_tau_nom-B_d_hat,CTRL.torque_limit);
previous=B_omega;
end

== matlab function V2/CoM Estimator/Algorithm ==
  settings: updateMethod=DISCRETE  sampleTime=CTRL.sample_time
  data: B_F_cmd input; B_c_hat output; B_d_hat input; B_c_filtered output; CTRL parameter
function [B_c_hat,B_c_filtered] = v2_moce(B_F_cmd,B_d_hat,CTRL)
%#codegen
persistent force_state estimate filtered
if isempty(force_state)
    force_state=zeros(2,3); estimate=CTRL.moce.initial_com(:); filtered=estimate;
end
dt=CTRL.sample_time;
[force_state,f,~]=v2_q(force_state,B_F_cmd,CTRL.moce.force_cutoff_rad_s,dt);
if ~CTRL.moce.enable
    estimate=CTRL.moce.initial_com(:);
elseif norm(f)>=CTRL.moce.min_force
    S=[0 -f(3) f(2);f(3) 0 -f(1);-f(2) f(1) 0];
    A=CTRL.nominal.inertia\S;
    rate=v2_bound(CTRL.moce.gamma(:).*(A'*B_d_hat),CTRL.moce.rate_limit);
    if ~CTRL.moce.estimate_z || norm(f(1:2))<CTRL.moce.min_horizontal_force, rate(3)=0; end
    estimate=v2_bound(estimate+dt*rate,CTRL.moce.offset_limit);
end
a=1;
if CTRL.moce.output_tau_s>0, a=1-exp(-dt/CTRL.moce.output_tau_s); end
filtered=filtered+a*(estimate-filtered);
B_c_hat=estimate; B_c_filtered=filtered;
end

== matlab function V2/Control Allocator/Algorithm ==
  settings: updateMethod=DISCRETE  sampleTime=CTRL.sample_time
  data: B_F_cmd input; thrust_cmd output; B_tau_cmd input; B_c_hat input; servo_angle input; servo_cmd output; CTRL parameter
function [thrust_cmd,servo_cmd] = v2_allocator(B_F_cmd,B_tau_cmd,B_c_hat,servo_angle,CTRL)
%#codegen
persistent yaw_lpf
if isempty(yaw_lpf), yaw_lpf=0; end
yaw_lpf=yaw_lpf+(1-exp(-2*pi*CTRL.allocator.yaw_split_cutoff_hz*CTRL.sample_time))*(B_tau_cmd(3)-yaw_lpf);
r=max(-CTRL.allocator.yaw_reaction_limit,min(CTRL.allocator.yaw_reaction_limit,B_tau_cmd(3)-yaw_lpf));
[p,d,reaction]=v2_rotors(servo_angle,CTRL.nominal.geometry,CTRL.nominal.propeller);
A1=zeros(4,4); A2=zeros(4,4);
for i=1:4
    moment=cross(p(:,i)-B_c_hat,d(:,i))+reaction(:,i);
    A1(:,i)=[moment(1:2);reaction(3,i);d(3,i)];
end
thrust_cmd=min(max(solve4(A1,[B_tau_cmd(1:2);r;B_F_cmd(3)],CTRL.allocator.regularization),0),CTRL.nominal.propeller.max_thrust);
for i=1:4
    tangent=CTRL.nominal.geometry.tangent(:,i)*thrust_cmd(i);
    moment=cross(p(:,i)-B_c_hat,tangent);
    A2(:,i)=[tangent(1:2);moment(3);CTRL.nominal.geometry.spin(i)*thrust_cmd(i)];
end
sine=solve4(A2,[B_F_cmd(1:2);B_tau_cmd(3)-r;0],CTRL.allocator.regularization);
servo_cmd=asin(min(max(sine,-sin(CTRL.nominal.servo_limit)),sin(CTRL.nominal.servo_limit)));
end
function x=solve4(A,b,lambda)
if rcond(A)>1e-10, x=A\b;
else, x=(A'*A+lambda*eye(4))\(A'*b); end
end

== matlab function V2/Rigid-Body Plant/Actuator Wrench Model/Algorithm ==
  data: thrust input; B_F_actual output; servo_angle input; B_tau_actual output; PLANT parameter
function [B_F_actual,B_tau_actual] = v2_wrench(thrust,servo_angle,PLANT)
%#codegen
[p,d,reaction]=v2_rotors(servo_angle,PLANT.geometry,PLANT.propeller);
B_F_actual=zeros(3,1); B_tau_actual=zeros(3,1);
for i=1:4
    f=thrust(i)*d(:,i);
    B_F_actual=B_F_actual+f;
    B_tau_actual=B_tau_actual+cross(p(:,i)-PLANT.derived.com,f)+thrust(i)*reaction(:,i);
end
end

== matlab function V2/Rigid-Body Plant/Rotational Dynamics/Euler rigid body equation/Algorithm ==
  data: B_tau_actual input; B_omega_dot output; B_omega input; PLANT parameter
function B_omega_dot = v2_rotation_dynamics(B_tau_actual,B_omega,PLANT)
%#codegen
J=PLANT.derived.inertia;
B_omega_dot=J\(B_tau_actual-cross(B_omega,J*B_omega));
end
